simulink model "unitTestCoordinateTransformations"  (R2018b)
settings: Solver=FixedStepDiscrete  StartTime=0.0  StopTime=10.0  FixedStep=.1  RelTol=1e-3  EnableMultiTasking=on
values from neighbouring files (symbols this model uses):
  alt = evalin('base','alt')    [unitTest_CoordinateTransformations.m]
  az_rad = evalin('base','az_rad')    [unitTest_CoordinateTransformations.m]
  azdot = randi(1e6,1)    [unitTest_CoordinateTransformations.m]
  el = atan(h/rh)    [unitTest_CoordinateTransformations.m]
  el_rad = evalin('base','el_rad')    [unitTest_CoordinateTransformations.m]
  eldot = randi(1e6,1)    [unitTest_CoordinateTransformations.m]
  h = evalin('base','h')    [unitTest_CoordinateTransformations.m]
  lat = evalin('base','lat')    [unitTest_CoordinateTransformations.m]
  lon = evalin('base','lon')    [unitTest_CoordinateTransformations.m]
  r = evalin('base', 'r')    [unitTest_CoordinateTransformations.m]
  rdot = randi(1e6,1)    [unitTest_CoordinateTransformations.m]
  theta = evalin('base','theta')    [unitTest_CoordinateTransformations.m]
  X = evalin('base','X')    [unitTest_CoordinateTransformations.m]
  x = evalin('base','x')    [unitTest_CoordinateTransformations.m]
  xdot = randi(1e6,1)    [unitTest_CoordinateTransformations.m]
  Y = evalin('base','Y')    [unitTest_CoordinateTransformations.m]
  y = evalin('base','y')    [unitTest_CoordinateTransformations.m]
  ydot = randi(1e6,1)    [unitTest_CoordinateTransformations.m]
  Z = evalin('base','Z')    [unitTest_CoordinateTransformations.m]
  z = evalin('base','z')    [unitTest_CoordinateTransformations.m]
  zdot = randi(1e6,1)    [unitTest_CoordinateTransformations.m]
libraries: ECEF2LLA x1, LLA2ECEF x1, cart2cyl x1, cart2sph_degas x1, cyl2cart x1, sph2cart x1
settings Model: Creator=AN21858  LastModifiedBy=BI28030
settings DataIOCC: LimitDataPoints=on  SaveFormat=Array
settings OptimizationCC: ExpressionDepthLimit=2147483647  LifeSpan=inf
settings DebuggingCC: UnderspecifiedInitializationDetection=Classic  MergeDetectMultiDrivingBlocksExec=none  SolverPrmCheckMsg=warning  StateNameClashWarn=warning  SFUnexpectedBacktrackingDiag=warning  SFNoUnconditionalDefaultTransitionDiag=warning  SFExecutionAtInitializationDiag=none
settings HardwareCC: ProdBitPerPointer=32  ProdBitPerSizeT=32  ProdBitPerPtrDiffT=32  ProdLargestAtomicFloat=None  ProdIntDivRoundTo=Undefined  ProdEndianess=Unspecified  ProdWordSize=32  ProdHWDeviceType=32-bit Generic
settings ModelReferenceCC: PropagateSignalLabelsOutOfModel=off
settings SFSimCC: SimUseLocalCustomCode=off
settings RTWCC: RTWUseLocalCustomCode=off
settings CodeAppCC: StateflowObjectComments=on
settings GRTTargetCC: TargetLangStandard=C89/C90 (ANSI)  GeneratePreprocessorConditionals=Disable all
settings ConfigComp: CovMetricSettings=dw  CovHtmlReporting=on  CovSaveCumulativeToWorkspaceVar=on  CovSaveSingleToWorkspaceVar=on  CovExternalEMLEnable=off

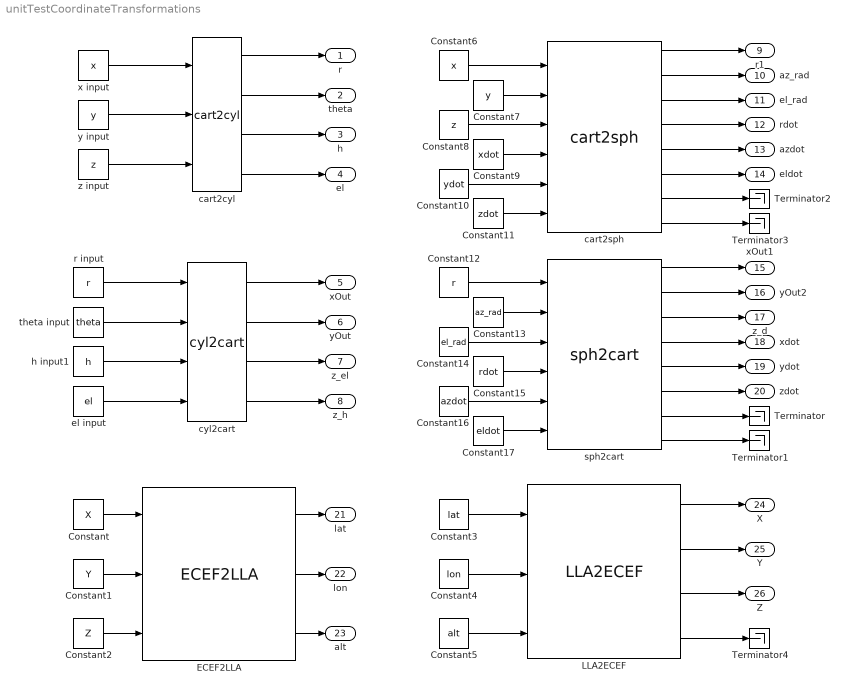
== system unitTestCoordinateTransformations ==
  Constant : Constant  Value=X
  Constant1 : Constant  Value=Y
  Constant10 : Constant  Value=ydot
  Constant11 : Constant  Value=zdot
  Constant12 : Constant  Value=r
  Constant13 : Constant  Value=az_rad
  Constant14 : Constant  Value=el_rad
  Constant15 : Constant  Value=rdot
  Constant16 : Constant  Value=azdot
  Constant17 : Constant  Value=eldot
  Constant2 : Constant  Value=Z
  Constant3 : Constant  Value=lat
  Constant4 : Constant  Value=lon
  Constant5 : Constant  Value=alt
  Constant6 : Constant  Value=x
  Constant7 : Constant  Value=y
  Constant8 : Constant  Value=z
  Constant9 : Constant  Value=xdot
  ECEF2LLA : ECEF2LLA/ECEF2LLA  a=6378137  b=6356752.31424518
  LLA2ECEF : LLA2ECEF/LLA2ECEF  a=6378137  b=6356752.31424518
  Terminator{,1..4} (5 alike) : Terminator
  cart2cyl : cart2cyl/cart2cyl
  cart2sph : cart2sph_degas/cart2sph  SystemSampleTime=-1
  cyl2cart : cyl2cart/cyl2cart
  el input : Constant  Value=el
  h input1 : Constant  Value=h
  r input : Constant  Value=r
  sph2cart : sph2cart/sph2cart  SystemSampleTime=-1
      settings: SourceProductName=CASSATTv6: Signals Library
  theta input : Constant  Value=theta
  x input : Constant  Value=x
  y input : Constant  Value=y
  z input : Constant  Value=z
  r : Outport
  theta : Outport  Port=2
  h : Outport  Port=3
  el : Outport  Port=4
  xOut : Outport  Port=5
  yOut : Outport  Port=6
  z_el : Outport  Port=7
  z_h : Outport  Port=8
  r1 : Outport  Port=9
  az_rad : Outport  Port=10
  el_rad : Outport  Port=11
  "rdot " : Outport  Port=12
  azdot : Outport  Port=13
  eldot : Outport  Port=14
  xOut1 : Outport  Port=15
  yOut2 : Outport  Port=16
  z_d : Outport  Port=17
  xdot : Outport  Port=18
  ydot : Outport  Port=19
  zdot : Outport  Port=20
  lat : Outport  Port=21
  lon : Outport  Port=22
  alt : Outport  Port=23
  X : Outport  Port=24
  Y : Outport  Port=25
  Z : Outport  Port=26
  wires:
  x input/1 -> cart2cyl/1
  y input/1 -> cart2cyl/2
  z input/1 -> cart2cyl/3
  cart2cyl/1 -> r/1
  cart2cyl/2 -> theta/1
  cart2cyl/3 -> h/1
  r input/1 -> cyl2cart/1
  theta input/1 -> cyl2cart/2
  h input1/1 -> cyl2cart/3
  cyl2cart/1 -> xOut/1
  cyl2cart/2 -> yOut/1
  cyl2cart/3 -> z_el/1
  cart2cyl/4 -> el/1
  el input/1 -> cyl2cart/4
  cyl2cart/4 -> z_h/1
  cart2sph/1 -> r1/1
  cart2sph/3 -> el_rad/1
  cart2sph/2 -> az_rad/1
  cart2sph/4 -> "rdot "/1
  cart2sph/5 -> azdot/1
  cart2sph/6 -> eldot/1
  cart2sph/7 -> Terminator2/1
  cart2sph/8 -> Terminator3/1
  sph2cart/1 -> xOut1/1
  sph2cart/2 -> yOut2/1
  sph2cart/3 -> z_d/1
  sph2cart/4 -> xdot/1
  sph2cart/5 -> ydot/1
  sph2cart/6 -> zdot/1
  sph2cart/7 -> Terminator/1
  sph2cart/8 -> Terminator1/1
  Constant/1 -> ECEF2LLA/1
  Constant2/1 -> ECEF2LLA/3
  Constant1/1 -> ECEF2LLA/2
  ECEF2LLA/1 -> lat/1
  ECEF2LLA/2 -> lon/1
  ECEF2LLA/3 -> alt/1
  LLA2ECEF/1 -> X/1
  LLA2ECEF/2 -> Y/1
  LLA2ECEF/3 -> Z/1
  LLA2ECEF/4 -> Terminator4/1
  Constant3/1 -> LLA2ECEF/1
  Constant5/1 -> LLA2ECEF/3
  Constant4/1 -> LLA2ECEF/2
  Constant6/1 -> cart2sph/1
  Constant7/1 -> cart2sph/2
  Constant8/1 -> cart2sph/3
  Constant9/1 -> cart2sph/4
  Constant10/1 -> cart2sph/5
  Constant11/1 -> cart2sph/6
  Constant12/1 -> sph2cart/1
  Constant13/1 -> sph2cart/2
  Constant14/1 -> sph2cart/3
  Constant15/1 -> sph2cart/4
  Constant16/1 -> sph2cart/5
  Constant17/1 -> sph2cart/6
